simulink library "delay_and_stop_when_change"  (R2024a)
settings: Solver=VariableStepAuto  StartTime=0.0  StopTime=10.0  RelTol=1e-3
settings Model: Creator=leona  LastModifiedBy=leona

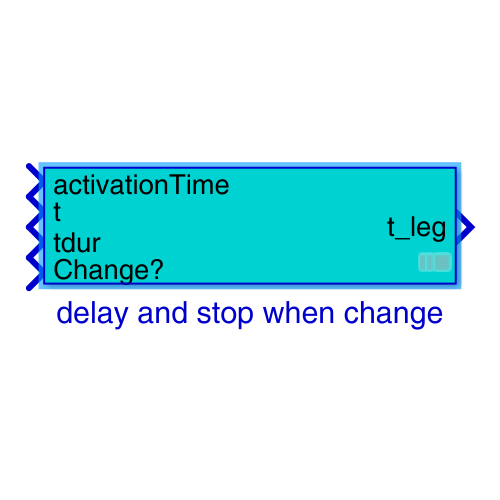
[thumbnail: Simulink's stored preview of the top-level diagram]
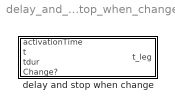
== system delay_and_stop_when_change ==
  delay and stop when change : Subsystem  mask{delay=0}

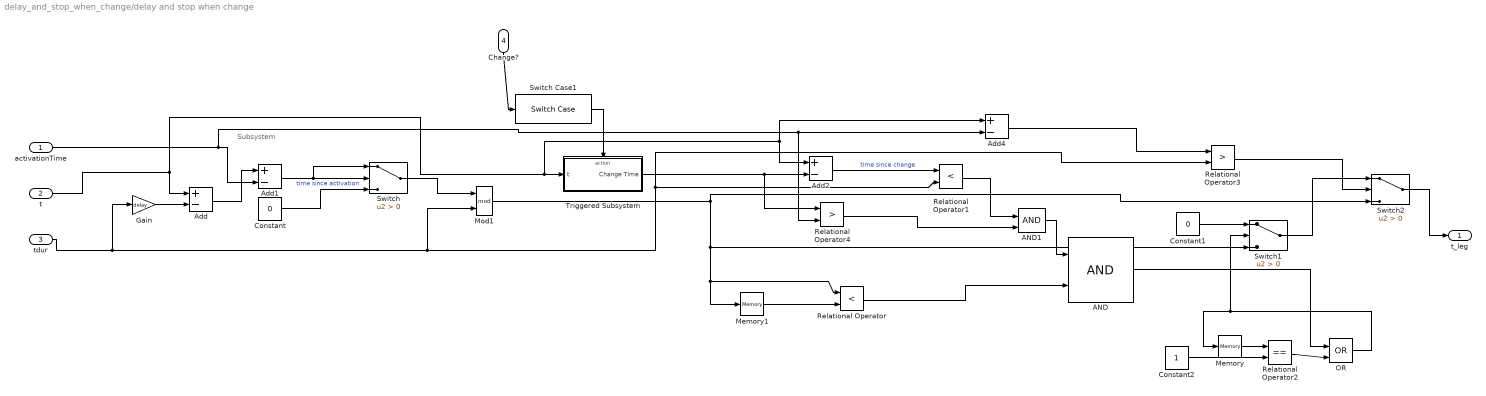
== system delay_and_stop_when_change/delay and stop when change ==
  note: Subsystem
  activationTime : Inport
  t : Inport  Port=2
  tdur : Inport  Port=3
  Change? : Inport  Port=4
  AND : Logic  IconShape=distinctive  AllPortsSameDT=off  OutDataTypeStr=boolean
  AND1 : Logic  IconShape=distinctive  AllPortsSameDT=off  OutDataTypeStr=boolean
  Add{,1..2,4} (4 alike) : Sum  Inputs=+-
  Constant : Constant  Value=0
  Constant1 : Constant  Value=0
  Constant2 : Constant
  Gain : Gain  Gain=delay
  Memory : Memory
  Memory1 : Memory
  Mod1 : Math  Operator=mod
  OR : Logic  Operator=OR  IconShape=distinctive  AllPortsSameDT=off  OutDataTypeStr=boolean
  Relational Operator : RelationalOperator  Operator=<  OutDataTypeStr=boolean  RndMeth=Simplest  InputSameDT=off
  Relational Operator1 : RelationalOperator  Operator=<  OutDataTypeStr=boolean  RndMeth=Simplest  InputSameDT=off
  Relational Operator2 : RelationalOperator  Operator===  OutDataTypeStr=boolean  RndMeth=Simplest  InputSameDT=off
  Relational Operator3 : RelationalOperator  Operator=>  OutDataTypeStr=boolean  RndMeth=Simplest  InputSameDT=off
  Relational Operator4 : RelationalOperator  Operator=>  OutDataTypeStr=boolean  RndMeth=Simplest  InputSameDT=off
  Switch : Switch  Criteria=u2 > Threshold  SaturateOnIntegerOverflow=off  InputSameDT=off
  Switch Case1 : SwitchCase  ShowDefaultCase=off
  Switch1 : Switch  Criteria=u2 > Threshold  SaturateOnIntegerOverflow=off  InputSameDT=off
  Switch2 : Switch  Criteria=u2 > Threshold  SaturateOnIntegerOverflow=off  InputSameDT=off
  Triggered Subsystem : Subsystem  TreatAsAtomicUnit=on
  t_leg : Outport
  wires:
  AND/1 -> OR/1
  OR/1 -> Memory/1, Switch1/2
  Memory/1 -> Relational Operator2/1
  Relational Operator/1 -> AND/2
  AND1/1 -> AND/1
  Relational Operator4/1 -> AND1/2
  activationTime/1 -> Add4/2, Relational Operator4/2, Add1/2
  Switch/1 -> Mod1/1
  Gain/1 -> Add/2
  t/1 -> Add2/1, Add4/1, Triggered Subsystem/1(t), Add/1
  Constant/1 -> Switch/3
  Add1/1 -> Switch/1, Switch/2  "time since activation"
  Add/1 -> Add1/1
  Switch Case1/1 -> Triggered Subsystem/Action
  Relational Operator1/1 -> AND1/1
  Constant1/1 -> Switch1/1
  Change?/1 -> Switch Case1/1
  Memory1/1 -> Relational Operator/2
  Switch1/1 -> Switch2/1
  Mod1/1 -> Switch2/3, Relational Operator/1, Memory1/1, Switch1/3
  Triggered Subsystem/1(Change Time) -> Add2/2, Relational Operator4/1
  Add2/1 -> Relational Operator1/1  "time since change"
  Relational Operator2/1 -> OR/2
  Constant2/1 -> Relational Operator2/2
  Switch2/1 -> t_leg/1
  Relational Operator3/1 -> Switch2/2
  tdur/1 -> Gain/1, Mod1/2, Relational Operator1/2, Relational Operator3/2
  Add4/1 -> Relational Operator3/1

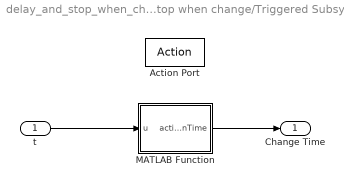
== system delay_and_stop_when_change/delay and stop when change/Triggered Subsystem ==
  t : Inport
  Action Port : ActionPort  InitializeStates=reset
  MATLAB Function : MATLAB Function  TreatAsAtomicUnit=on
  Change Time : Outport
  wires:
  MATLAB Function/1(activationTime) -> Change Time/1
  t/1 -> MATLAB Function/1(u)

== matlab function delay_and_stop_when_change/delay and stop when change/Triggered Subsystem/MATLAB Function ==
  data: u input; activationTime output
function activationTime = getActivationTime(u)
    persistent t_start
    if isempty(t_start)
        t_start = u;
    end
    activationTime = t_start;
end
